simulink model "tesssst"  (R2015a)
settings: Solver=ode3  StartTime=0.0  StopTime=10.0  FixedStep=0.001  RelTol=1e-3
values from neighbouring files (symbols this model uses):
  anpha_0 = 5    [ANN_params.m]    (also in furuta.m)
  K = lqr(A,B,Q,r)    [lqr_pen.m]
  theta_0 = 0    [ANN_params.m]    (also in furuta.m)
settings Model: Creator=chech  LastModifiedBy=chech

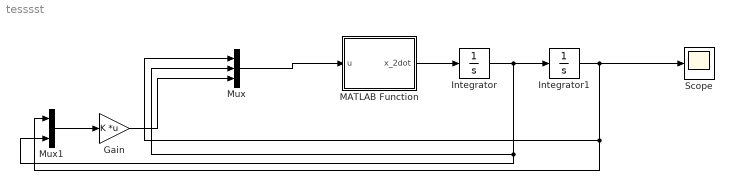
== system tesssst ==
  Gain : Gain  Gain=K  Multiplication=Matrix(K*u)
  Integrator : Integrator  InitialCondition=[0;0]
  Integrator1 : Integrator  InitialCondition=[theta_0;anpha_0]
  MATLAB Function : MATLAB Function  TreatAsAtomicUnit=on
  Mux : Mux  Inputs=3
  Mux1 : Mux  Inputs=2
  Scope : Scope
      settings: YMin=-4e+06  YMax=500000
  wires:
  MATLAB Function/1(x_2dot) -> Integrator/1
  Integrator/1 -> Mux1/2, Mux/2, Integrator1/1
  Integrator1/1 -> Scope/1, Mux1/1, Mux/1
  Gain/1 -> Mux/3
  Mux/1 -> MATLAB Function/1(u)
  Mux1/1 -> Gain/1

== matlab function tesssst/MATLAB Function ==
  data: u input size=5; x_2dot output size=2
function x_2dot = fcn(u)
%#codegen
m1=0.078;
L0=0.157;
L1=0.133;
J0=4.4*10^(-3);
J1=5.5026*10^(-4);
beta0 = 5.8*10^(-4);
beta1 = 1.4142*10^(-3);
g = 9.81;
f1_num = m1*L0*L1*cos(u(2))*(0.5*m1*L1^2*sin(2*u(2))*u(3)^2+m1*g*L1*sin(u(2))-beta1*u(4))-(m1*L1^2+J1)*(m1*L1^2*sin(2*u(2))*u(3)*u(4)+m1*L0*L1*sin(u(2))*u(4)^2-u(5)+beta0*u(3));
f2_num = (m1*L0^2+m1*L1^2*sin(u(2))^2+J0)*(0.5*m1*L1^2*sin(2*u(2))*u(3)^2+m1*g*L1*sin(u(2))-beta1*u(4))-m1*L0*L1*cos(u(2))*(m1*L1^2*sin(2*u(2))*u(3)*u(4)+m1*L0*L1*sin(u(2))*u(4)^2-u(5)+beta0*u(3));
denta = J0*J1+m1^2*L1^4*sin(u(2))^2+m1^2*L0^2*L1^2+J0*m1*L1^2+J1*m1*L0^2+J1*m1*L1^2*sin(u(2))^2-m1^2*L0^2*L1^2*cos(u(2))^2;
x_2dot = [f1_num/denta;
    f2_num/denta];
